simulink model "pct23_lab"  (R2020b)
settings: Solver=VariableStepAuto  StartTime=0.0  StopTime=inf  RelTol=1e-3
libraries: pct23_lib x1
settings Model: EnablePacing=on  Creator=MK  LastModifiedBy=lgalc
settings DataIOCC: ReturnWorkspaceOutputs=off
settings DebuggingCC: ArithmeticOperatorsInVariantConditions=warning
settings SFSimCC: CustomCodeUndefinedFunction=UseInterfaceOnly

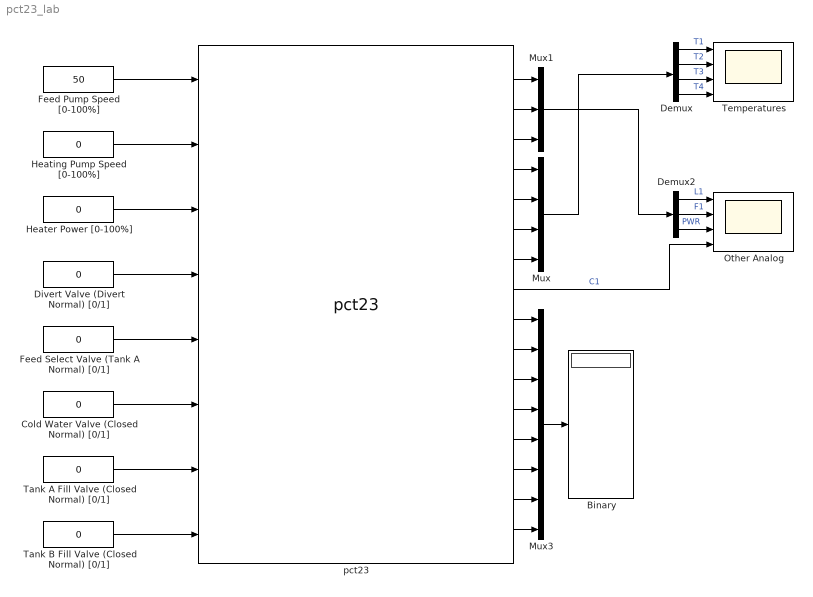
== system pct23_lab ==
  Binary : Display
  Cold Water Valve (Closed Normal) [0/1] : Constant  Value=0
  Demux : Demux
  Demux2 : Demux  Outputs=3
  Divert Valve (Divert Normal) [0/1] : Constant  Value=0
  Feed Pump Speed [0-100%] : Constant  Value=50
  Feed Select Valve (Tank A Normal) [0/1] : Constant  Value=0
  Heater Power [0-100%] : Constant  Value=0
  Heating Pump Speed [0-100%] : Constant  Value=0
  Mux : Mux
  Mux1 : Mux  Inputs=3
  Mux3 : Mux  Inputs=8
  Other Analog : Scope  NumInputPorts=4
  Tank A Fill Valve (Closed Normal) [0/1] : Constant  Value=0
  Tank B Fill Valve (Closed Normal) [0/1] : Constant  Value=0
  Temperatures : Scope  NumInputPorts=4
  pct23 : pct23_lib/pct23  SystemSampleTime=-1  VariantActivationTime=update diagram  Latency=0  AutoFrameSizeCalculation=off
  wires:
  Feed Pump Speed [0-100%]/1 -> pct23/1
  Heating Pump Speed [0-100%]/1 -> pct23/2
  Tank B Fill Valve (Closed Normal) [0/1]/1 -> pct23/8
  Tank A Fill Valve (Closed Normal) [0/1]/1 -> pct23/7
  Cold Water Valve (Closed Normal) [0/1]/1 -> pct23/6
  Divert Valve (Divert Normal) [0/1]/1 -> pct23/4
  Heater Power [0-100%]/1 -> pct23/3
  Feed Select Valve (Tank A Normal) [0/1]/1 -> pct23/5
  pct23/4 -> Mux/1
  pct23/5 -> Mux/2
  pct23/6 -> Mux/3
  pct23/7 -> Mux/4
  Mux/1 -> Demux/1
  Demux/2 -> Temperatures/2  "T2"
  Demux/4 -> Temperatures/4  "T4"
  Demux/3 -> Temperatures/3  "T3"
  Demux/1 -> Temperatures/1  "T1"
  Demux2/1 -> Other Analog/1  "L1"
  Demux2/2 -> Other Analog/2  "F1"
  Demux2/3 -> Other Analog/3  "PWR"
  Mux1/1 -> Demux2/1
  pct23/8 -> Other Analog/4  "C1"
  pct23/1 -> Mux1/1
  pct23/2 -> Mux1/2
  pct23/3 -> Mux1/3
  Mux3/1 -> Binary/1
  pct23/9 -> Mux3/1
  pct23/10 -> Mux3/2
  pct23/11 -> Mux3/3
  pct23/12 -> Mux3/4
  pct23/13 -> Mux3/5
  pct23/14 -> Mux3/6
  pct23/15 -> Mux3/7
  pct23/16 -> Mux3/8
